simulink model "Estimador_DB_Caso_2_Bis"  (R2023a)
settings: Solver=VariableStepAuto  StartTime=0.0  StopTime=7  MaxStep=0.001  MinStep=0.0001  RelTol=1e-3
undefined symbols (not defined in the file): g, g0, K, Ke, l, M, m
settings Model: Creator=54115  LastModifiedBy=franc
settings SolverCC: AlgebraicLoopSolver=TrustRegion
settings DebuggingCC: UnconnectedInputMsg=warning  UnconnectedOutputMsg=warning  UnconnectedLineMsg=warning
settings ModelReferenceCC: EnableRefExpFcnMdlSchedulingChecks=on

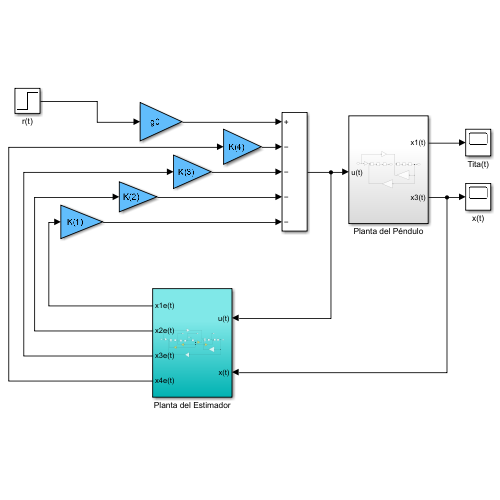
[thumbnail: Simulink's stored preview of the top-level diagram]
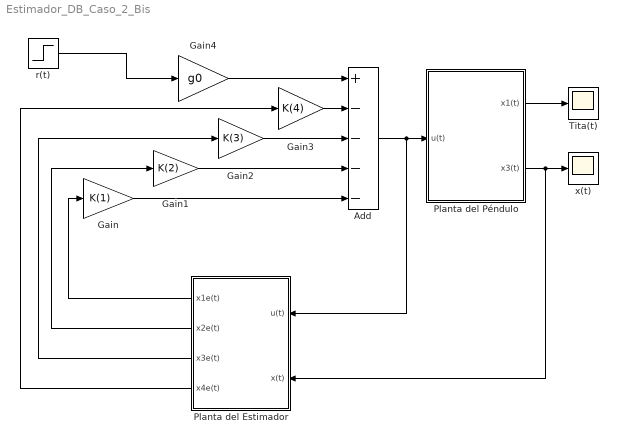
== system Estimador_DB_Caso_2_Bis ==
  Add : Sum  Inputs=+----
  Gain : Gain  Gain=K(1)
  Gain1 : Gain  Gain=K(2)
  Gain2 : Gain  Gain=K(3)
  Gain3 : Gain  Gain=K(4)
  Gain4 : Gain  Gain=g0
  Planta del Estimador : Subsystem
  Planta del Péndulo : Subsystem
  "Tita(t) " : Scope
  r(t) : Step  Time=0  SampleTime=0
  x(t) : Scope
  wires:
  Planta del Péndulo/2(x3(t)) -> Planta del Estimador/2(x(t)), x(t)/1
  Gain/1 -> Add/5
  Gain1/1 -> Add/4
  Gain2/1 -> Add/3
  Gain3/1 -> Add/2
  Gain4/1 -> Add/1
  r(t)/1 -> Gain4/1
  Add/1 -> Planta del Péndulo/1(u(t)), Planta del Estimador/1(u(t))
  Planta del Péndulo/1(x1(t)) -> "Tita(t) "/1
  Planta del Estimador/4(x4e(t)) -> Gain3/1
  Planta del Estimador/3(x3e(t)) -> Gain2/1
  Planta del Estimador/2(x2e(t)) -> Gain1/1
  Planta del Estimador/1(x1e(t)) -> Gain/1

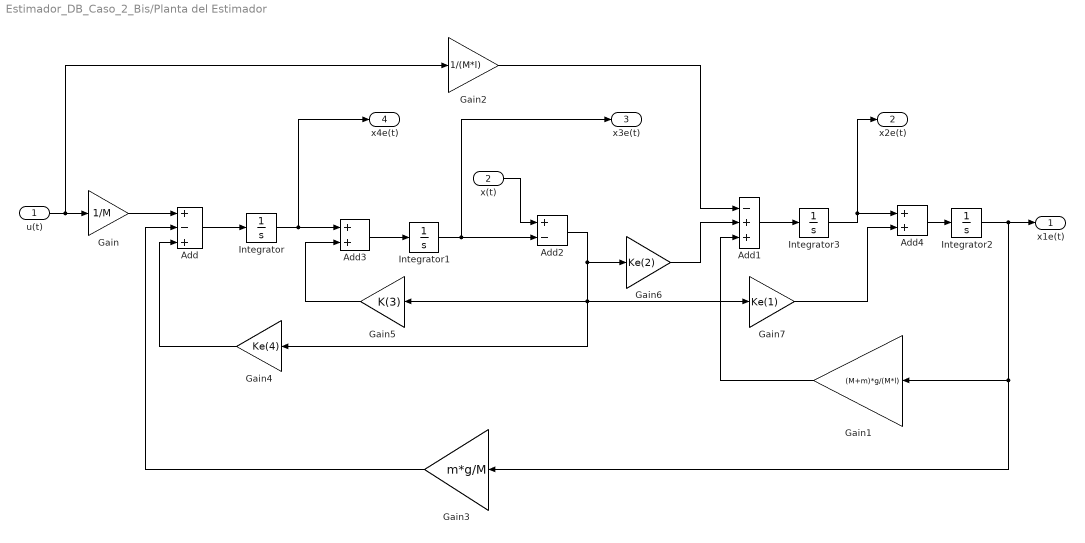
== system Estimador_DB_Caso_2_Bis/Planta del Estimador ==
  u(t) : Inport
  x(t) : Inport  Port=2
  Add : Sum  Inputs=+-+
  Add1 : Sum  Inputs=-++
  Add2 : Sum  Inputs=+-
  Add3 : Sum
  Add4 : Sum
  Gain : Gain  Gain=1/M
  Gain1 : Gain  Gain=(M+m)*g/(M*l)
  Gain2 : Gain  Gain=1/(M*l)
  Gain3 : Gain  Gain=m*g/M
  Gain4 : Gain  Gain=Ke(4)
  Gain5 : Gain  Gain=K(3)
  Gain6 : Gain  Gain=Ke(2)
  Gain7 : Gain  Gain=Ke(1)
  Integrator{,1..3} (4 alike) : Integrator
  x1e(t) : Outport
  x2e(t) : Outport  Port=2
  x3e(t) : Outport  Port=3
  x4e(t) : Outport  Port=4
  wires:
  Add/1 -> Integrator/1
  Integrator/1 -> Add3/1, x4e(t)/1
  Integrator1/1 -> Add2/2, x3e(t)/1
  Integrator2/1 -> x1e(t)/1, Gain1/1, Gain3/1
  u(t)/1 -> Gain/1, Gain2/1
  Integrator3/1 -> x2e(t)/1, Add4/1
  Gain/1 -> Add/1
  Add1/1 -> Integrator3/1
  Gain2/1 -> Add1/1
  Gain3/1 -> Add/2
  x(t)/1 -> Add2/1
  Gain4/1 -> Add/3
  Add2/1 -> Gain6/1, Gain7/1, Gain4/1, Gain5/1
  Add3/1 -> Integrator1/1
  Gain5/1 -> Add3/2
  Gain1/1 -> Add1/3
  Gain6/1 -> Add1/2
  Add4/1 -> Integrator2/1
  Gain7/1 -> Add4/2

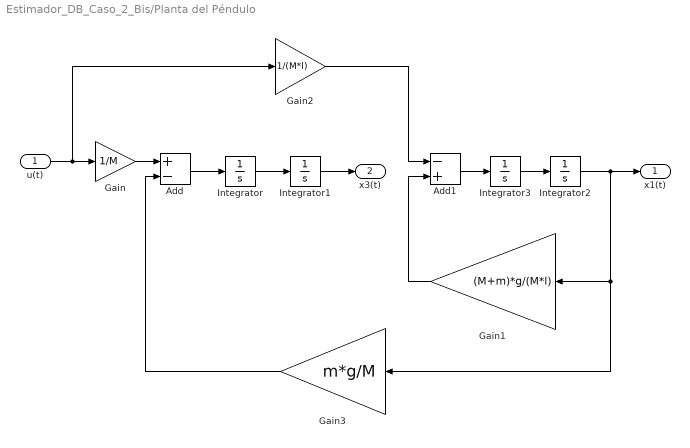
== system Estimador_DB_Caso_2_Bis/Planta del Péndulo ==
  u(t) : Inport
  Add : Sum  Inputs=+-
  Add1 : Sum  Inputs=-+
  Gain : Gain  Gain=1/M
  Gain1 : Gain  Gain=(M+m)*g/(M*l)
  Gain2 : Gain  Gain=1/(M*l)
  Gain3 : Gain  Gain=m*g/M
  Integrator{,1..3} (4 alike) : Integrator
  x1(t) : Outport
  x3(t) : Outport  Port=2
  wires:
  Add1/1 -> Integrator3/1
  Gain1/1 -> Add1/2
  Gain/1 -> Add/1
  Integrator/1 -> Integrator1/1
  Integrator1/1 -> x3(t)/1
  Gain2/1 -> Add1/1
  Gain3/1 -> Add/2
  Integrator3/1 -> Integrator2/1
  Integrator2/1 -> x1(t)/1, Gain3/1, Gain1/1
  u(t)/1 -> Gain2/1, Gain/1
  Add/1 -> Integrator/1
